simulink model "Phase_Control_K1_closed"  (R2018b)
settings: Solver=VariableStepAuto  StartTime=0.0  StopTime=200  RelTol=1e-3
values from neighbouring files (symbols this model uses):
  alpha = 0.5736    [constants.m]
  c_damp = 0.00495    [constants.m]
  delay = 0.8    [constants.m]
  dis_torque = 0.001    [constants.m]
  in_nu = 0.0001    [constants.m]
  J_r = 0.0004    [constants.m]
  J_s = 31.38    [constants.m]
  noise = 10^-9    (= 1e-09)    [constants.m]
  T_sat = 0.05    [constants.m]
  w_mode = 2.6268    [constants.m]
  w_sat = 2800*2*pi/60    (= 293.215314335)    [constants.m]
settings Model: Creator=Yavuz  LastModifiedBy=Yavuz
settings DebuggingCC: AlgebraicLoopMsg=none

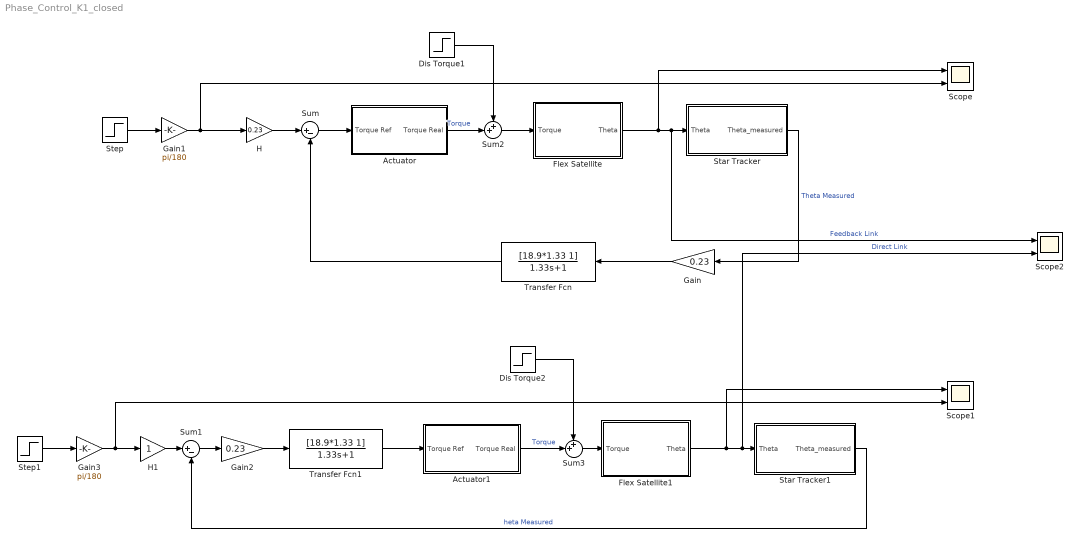
== system Phase_Control_K1_closed ==
  Actuator : Subsystem
  Actuator1 : Subsystem
  Dis Torque1 : Step  Time=100  After=dis_torque  SampleTime=0
  Dis Torque2 : Step  Time=100  After=dis_torque  SampleTime=0
  Flex Satellite : Subsystem
  Flex Satellite1 : Subsystem
  Gain : Gain  Gain=0.23
  Gain1 : Gain  Gain=pi/180
  Gain2 : Gain  Gain=0.23
  Gain3 : Gain  Gain=pi/180
  H : Gain  Gain=0.23
  H1 : Gain
  Scope : Scope  NumInputPorts=2
  Scope1 : Scope  NumInputPorts=2
  Scope2 : Scope  NumInputPorts=2
  Star Tracker : Subsystem
  Star Tracker1 : Subsystem
  Step : Step  Time=0  After=0.5  SampleTime=0
  Step1 : Step  Time=0  After=0.5  SampleTime=0
  Sum : Sum  Inputs=|+-
  Sum1 : Sum  Inputs=|+-
  Sum2 : Sum  Inputs=++|
  Sum3 : Sum  Inputs=++|
  Transfer Fcn : TransferFcn  Numerator=[18.9*1.33 1]  Denominator=[1.33 1]
  Transfer Fcn1 : TransferFcn  Numerator=[18.9*1.33 1]  Denominator=[1.33 1]
  wires:
  Flex Satellite/1(Theta) -> Scope/1, Scope2/1, Star Tracker/1(Theta)  "Feedback Link"
  Star Tracker/1(Theta_measured) -> Gain/1  "Theta Measured"
  Gain/1 -> Transfer Fcn/1
  Transfer Fcn/1 -> Sum/2
  Gain1/1 -> Scope/2, H/1
  Sum/1 -> Actuator/1(Torque Ref)
  Step/1 -> Gain1/1
  H/1 -> Sum/1
  Flex Satellite1/1(Theta) -> Scope1/1, Scope2/2, Star Tracker1/1(Theta)  "Direct Link"
  Gain2/1 -> Transfer Fcn1/1
  Transfer Fcn1/1 -> Actuator1/1(Torque Ref)
  Gain3/1 -> Scope1/2, H1/1
  Step1/1 -> Gain3/1
  H1/1 -> Sum1/1
  Sum1/1 -> Gain2/1
  Star Tracker1/1(Theta_measured) -> Sum1/2  "heta Measured"
  Actuator/1(Torque Real) -> Sum2/2  "Torque"
  Sum2/1 -> Flex Satellite/1(Torque)
  Dis Torque1/1 -> Sum2/1
  Actuator1/1(Torque Real) -> Sum3/2  "Torque"
  Sum3/1 -> Flex Satellite1/1(Torque)
  Dis Torque2/1 -> Sum3/1

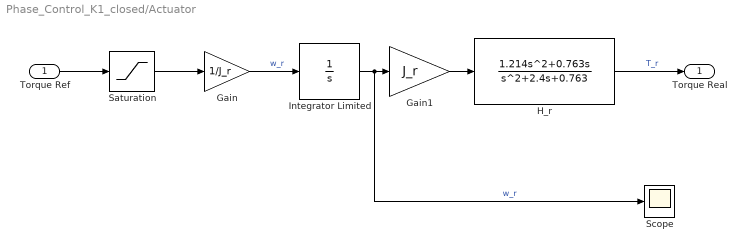
== system Phase_Control_K1_closed/Actuator ==
  Torque Ref : Inport
  Gain : Gain  Gain=1/J_r
  Gain1 : Gain  Gain=J_r
  H_r : TransferFcn  Numerator=[1.214 0.763 0]  Denominator=[1 2.4 0.763]
  Integrator Limited : Integrator  LimitOutput=on  UpperSaturationLimit=w_sat  LowerSaturationLimit=-w_sat
  Saturation : Saturate  UpperLimit=T_sat  LowerLimit=-T_sat
  Scope : Scope
  Torque Real : Outport
  wires:
  Torque Ref/1 -> Saturation/1
  Gain1/1 -> H_r/1
  H_r/1 -> Torque Real/1  "T_r"
  Gain/1 -> Integrator Limited/1  "w_r"
  Saturation/1 -> Gain/1
  Integrator Limited/1 -> Scope/1, Gain1/1  "w_r"

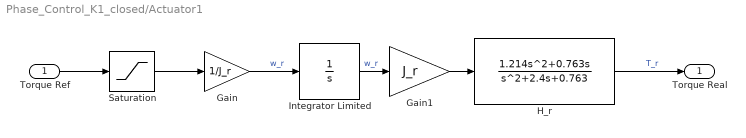
== system Phase_Control_K1_closed/Actuator1 ==
  Torque Ref : Inport
  Gain : Gain  Gain=1/J_r
  Gain1 : Gain  Gain=J_r
  H_r : TransferFcn  Numerator=[1.214 0.763 0]  Denominator=[1 2.4 0.763]
  Integrator Limited : Integrator  LimitOutput=on  UpperSaturationLimit=w_sat  LowerSaturationLimit=-w_sat
  Saturation : Saturate  UpperLimit=T_sat  LowerLimit=-T_sat
  Torque Real : Outport
  wires:
  Torque Ref/1 -> Saturation/1
  Gain1/1 -> H_r/1
  H_r/1 -> Torque Real/1  "T_r"
  Gain/1 -> Integrator Limited/1  "w_r"
  Saturation/1 -> Gain/1
  Integrator Limited/1 -> Gain1/1  "w_r"

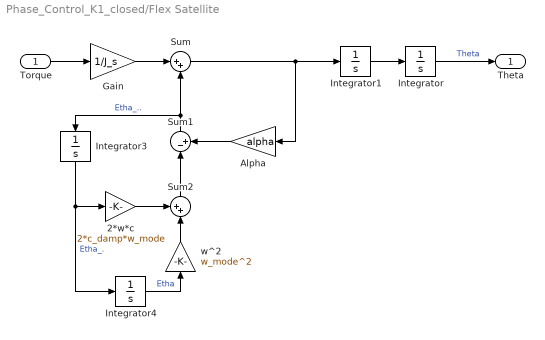
== system Phase_Control_K1_closed/Flex Satellite ==
  Torque : Inport
  2*w*c : Gain  Gain=2*c_damp*w_mode
  Alpha : Gain  Gain=alpha
  Gain : Gain  Gain=1/J_s
  Integrator : Integrator
  Integrator1 : Integrator
  Integrator3 : Integrator
  Integrator4 : Integrator  InitialCondition=in_nu
  Sum : Sum  Inputs=|++
  Sum1 : Sum  Inputs=|-+
  Sum2 : Sum  Inputs=++|
  w^2 : Gain  Gain=w_mode^2
  Theta : Outport
  wires:
  Sum/1 -> Integrator1/1, Alpha/1
  Sum1/1 -> Integrator3/1, Sum/2  "Etha_.."
  Gain/1 -> Sum/1
  Integrator1/1 -> Integrator/1
  Integrator3/1 -> Integrator4/1, 2*w*c/1  "Etha_."
  Sum2/1 -> Sum1/1
  Torque/1 -> Gain/1
  2*w*c/1 -> Sum2/1
  Integrator/1 -> Theta/1  "Theta"
  w^2/1 -> Sum2/2
  Integrator4/1 -> w^2/1  "Etha"
  Alpha/1 -> Sum1/2

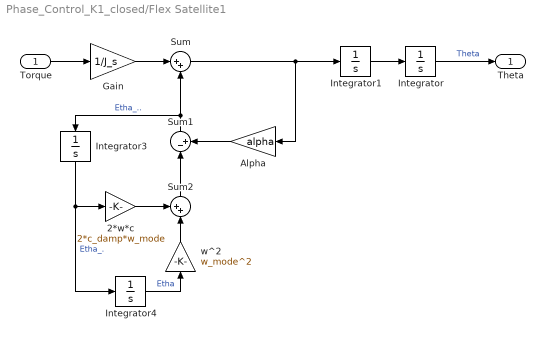
== system Phase_Control_K1_closed/Flex Satellite1 ==
  Torque : Inport
  2*w*c : Gain  Gain=2*c_damp*w_mode
  Alpha : Gain  Gain=alpha
  Gain : Gain  Gain=1/J_s
  Integrator : Integrator
  Integrator1 : Integrator
  Integrator3 : Integrator
  Integrator4 : Integrator  InitialCondition=in_nu
  Sum : Sum  Inputs=|++
  Sum1 : Sum  Inputs=|-+
  Sum2 : Sum  Inputs=++|
  w^2 : Gain  Gain=w_mode^2
  Theta : Outport
  wires:
  Sum/1 -> Integrator1/1, Alpha/1
  Sum1/1 -> Integrator3/1, Sum/2  "Etha_.."
  Gain/1 -> Sum/1
  Integrator1/1 -> Integrator/1
  Integrator3/1 -> Integrator4/1, 2*w*c/1  "Etha_."
  Sum2/1 -> Sum1/1
  Torque/1 -> Gain/1
  2*w*c/1 -> Sum2/1
  Integrator/1 -> Theta/1  "Theta"
  w^2/1 -> Sum2/2
  Integrator4/1 -> w^2/1  "Etha"
  Alpha/1 -> Sum1/2

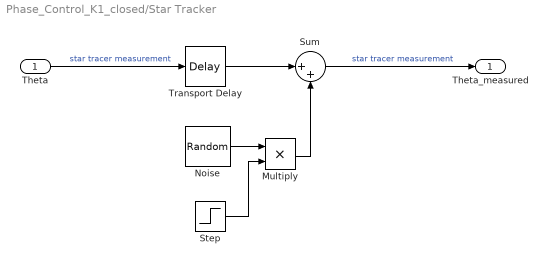
== system Phase_Control_K1_closed/Star Tracker ==
  Theta : Inport
  Multiply : Product
  Noise : RandomNumber  Variance=noise  SampleTime=0.1
  Step : Step  Time=160  SampleTime=0
  Sum : Sum  Inputs=|++
  Transport Delay : TransportDelay  DelayTime=delay
  Theta_measured : Outport
  wires:
  Theta/1 -> Transport Delay/1  "star tracer measurement"
  Noise/1 -> Multiply/1
  Step/1 -> Multiply/2
  Multiply/1 -> Sum/2
  Transport Delay/1 -> Sum/1
  Sum/1 -> Theta_measured/1  "star tracer measurement"

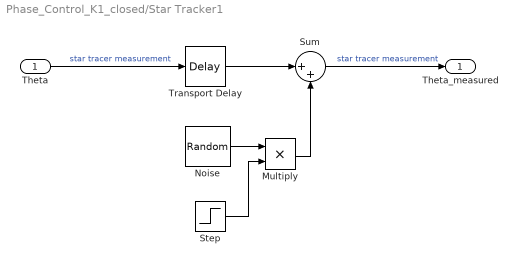
== system Phase_Control_K1_closed/Star Tracker1 ==
  Theta : Inport
  Multiply : Product
  Noise : RandomNumber  Variance=noise  SampleTime=0.1
  Step : Step  Time=160  SampleTime=0
  Sum : Sum  Inputs=|++
  Transport Delay : TransportDelay  DelayTime=delay
  Theta_measured : Outport
  wires:
  Theta/1 -> Transport Delay/1  "star tracer measurement"
  Noise/1 -> Multiply/1
  Step/1 -> Multiply/2
  Multiply/1 -> Sum/2
  Transport Delay/1 -> Sum/1
  Sum/1 -> Theta_measured/1  "star tracer measurement"
